simulink model "PMSM_NFLUX_v1_0"  (R2023b)
settings: Solver=FixedStepAuto  StartTime=0.0  StopTime=10.0  FixedStep=0.0001  RelTol=1e-3
values from neighbouring files (symbols this model uses):
  B = 8.0E-5    [PMSM_NFLUX.sldd]    (also in PMSM_NFLUX_backup_before_Simulink_RsStandstillID_20260617_154804.sldd; init_PMSM_NFLUX.m = single(8e-5))
  curr_d_ki = 35.0    [PMSM_NFLUX.sldd]    (also in PMSM_NFLUX_backup_before_Simulink_RsStandstillID_20260617_154804.sldd; init_PMSM_NFLUX.m = 35)
  curr_d_kp = 0.017    [PMSM_NFLUX.sldd]    (also in PMSM_NFLUX_backup_before_Simulink_RsStandstillID_20260617_154804.sldd; init_PMSM_NFLUX.m = 0.017)
  curr_q_ki = 35.0    [PMSM_NFLUX.sldd]    (also in PMSM_NFLUX_backup_before_Simulink_RsStandstillID_20260617_154804.sldd; init_PMSM_NFLUX.m = 35)
  curr_q_kp = 0.017    [PMSM_NFLUX.sldd]    (also in PMSM_NFLUX_backup_before_Simulink_RsStandstillID_20260617_154804.sldd; init_PMSM_NFLUX.m = 0.017)
  flux = 0.016884    [PMSM_NFLUX.sldd]    (also in PMSM_NFLUX_backup_before_Simulink_RsStandstillID_20260617_154804.sldd; init_PMSM_NFLUX.m = single(0.016884))
  Gamma = 100000.0    [PMSM_NFLUX.sldd]    (also in PMSM_NFLUX_backup_before_Simulink_RsStandstillID_20260617_154804.sldd; init_PMSM_NFLUX.m = single(100000.0))
  iq_handover = 0.4    [PMSM_NFLUX.sldd]    (also in PMSM_NFLUX_backup_before_Simulink_RsStandstillID_20260617_154804.sldd; init_PMSM_NFLUX.m = single(0.4))
  iq_ref_slew_down = 2.0    [PMSM_NFLUX.sldd]    (also in PMSM_NFLUX_backup_before_Simulink_RsStandstillID_20260617_154804.sldd; init_PMSM_NFLUX.m = single(2.0))
  iq_ref_slew_up = 5.0    [PMSM_NFLUX.sldd]    (also in PMSM_NFLUX_backup_before_Simulink_RsStandstillID_20260617_154804.sldd; init_PMSM_NFLUX.m = single(5.0))
  J = 7.5E-5    [PMSM_NFLUX.sldd]    (also in PMSM_NFLUX_backup_before_Simulink_RsStandstillID_20260617_154804.sldd; init_PMSM_NFLUX.m = single(75e-6))
  L = 0.00535    [PMSM_NFLUX.sldd]    (also in PMSM_NFLUX_backup_before_Simulink_RsStandstillID_20260617_154804.sldd; init_PMSM_NFLUX.m = single(0.00535))
  load_torque = 0.0    [PMSM_NFLUX.sldd]    (also in PMSM_NFLUX_backup_before_Simulink_RsStandstillID_20260617_154804.sldd; init_PMSM_NFLUX.m = single(0.0))
  LPF_K = 0.003    [PMSM_NFLUX.sldd]    (also in PMSM_NFLUX_backup_before_Simulink_RsStandstillID_20260617_154804.sldd; init_PMSM_NFLUX.m = single(0.003))
  PLL_Ki = 2500.0    [PMSM_NFLUX.sldd]    (also in PMSM_NFLUX_backup_before_Simulink_RsStandstillID_20260617_154804.sldd; init_PMSM_NFLUX.m = single(2500))
  PLL_Kp = 212.1    [PMSM_NFLUX.sldd]    (also in PMSM_NFLUX_backup_before_Simulink_RsStandstillID_20260617_154804.sldd; init_PMSM_NFLUX.m = single(212.1))
  PLL_OmegaLimit = 6283.18555    [PMSM_NFLUX.sldd]    (also in PMSM_NFLUX_backup_before_Simulink_RsStandstillID_20260617_154804.sldd; init_PMSM_NFLUX.m = single(2.0 * pi * 1000.0))
  Pn = 4.0    [PMSM_NFLUX.sldd]    (also in PMSM_NFLUX_backup_before_Simulink_RsStandstillID_20260617_154804.sldd; init_PMSM_NFLUX.m = single(4))
  PWM_HalfPeriod = 8000.0    [PMSM_NFLUX.sldd]    (also in PMSM_NFLUX_backup_before_Simulink_RsStandstillID_20260617_154804.sldd; init_PMSM_NFLUX.m = single(8000))
  Rs = 6.97    [PMSM_NFLUX.sldd]    (also in PMSM_NFLUX_backup_before_Simulink_RsStandstillID_20260617_154804.sldd; init_PMSM_NFLUX.m = single(6.97))
  spd_ki = 0.00165394868    [PMSM_NFLUX.sldd]    (also in PMSM_NFLUX_backup_before_Simulink_RsStandstillID_20260617_154804.sldd; init_PMSM_NFLUX.m = (B * speed_bw / Kt) * rpm_to_radps)
  spd_kp = 0.001550577    [PMSM_NFLUX.sldd]    (also in PMSM_NFLUX_backup_before_Simulink_RsStandstillID_20260617_154804.sldd; init_PMSM_NFLUX.m = (J * speed_bw / Kt) * rpm_to_radps)
  theta_handover_slew_limit = 5.0    [PMSM_NFLUX.sldd]    (also in PMSM_NFLUX_backup_before_Simulink_RsStandstillID_20260617_154804.sldd; init_PMSM_NFLUX.m = single(5.0))
  Tpwm = 16000.0    [PMSM_NFLUX.sldd]    (also in PMSM_NFLUX_backup_before_Simulink_RsStandstillID_20260617_154804.sldd; init_PMSM_NFLUX.m = 2 * PWM_HalfPeriod)
  Ts = 0.0001    [PMSM_NFLUX.sldd]    (also in PMSM_NFLUX_backup_before_Simulink_RsStandstillID_20260617_154804.sldd; init_PMSM_NFLUX.m = 0.0001)
  Udc = 24.0    [PMSM_NFLUX.sldd]    (also in PMSM_NFLUX_backup_before_Simulink_RsStandstillID_20260617_154804.sldd; init_PMSM_NFLUX.m = single(24.0))
undefined symbols (not defined in the file or in its folder): DiscIntNeverNeededParam, magnitude, sigbuilder_block
libraries: slpidlib x4, mcbplantlib x1, simulink x1, autolibpmsmexterior x1
(part 1 of 2)
settings Model: Creator=Administrator  LastModifiedBy=Kypuro

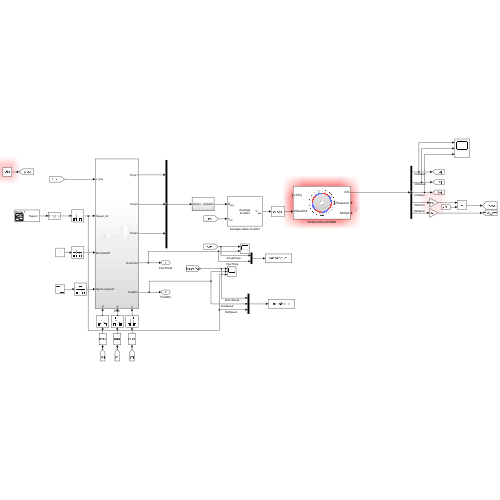
[thumbnail: Simulink's stored preview of the top-level diagram]
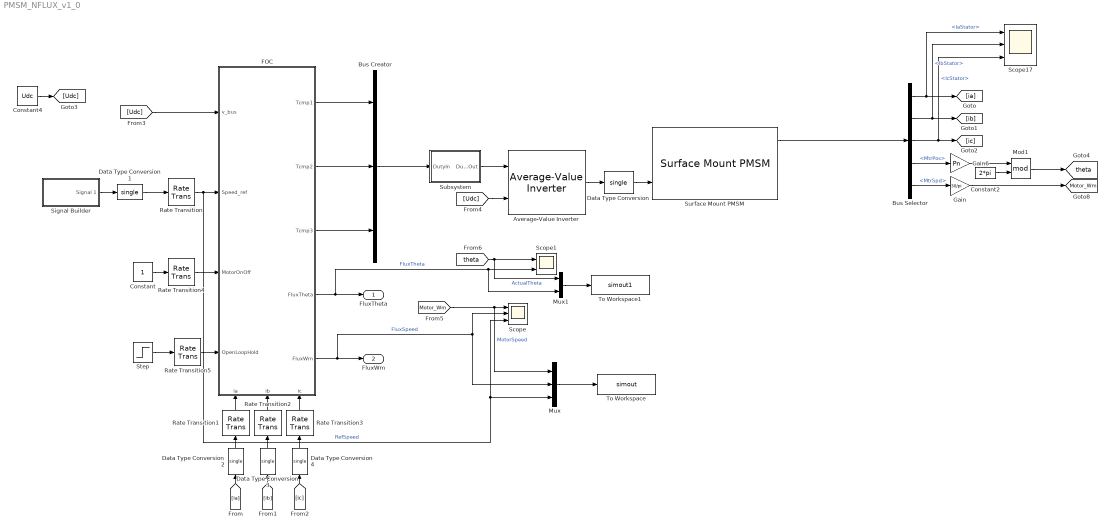
== system PMSM_NFLUX_v1_0 ==
  Average-Value Inverter : mcbplantlib/Average-Value Inverter
  Bus Creator : BusCreator  Inputs=3
  Bus Selector : BusSelector  OutputSignals=IaStator,IbStator,IcStator,MtrPos,MtrSpd
  Constant : Constant
  Constant2 : Constant  Value=2*pi  OutDataTypeStr=single
  Constant4 : Constant  Value=Udc  OutDataTypeStr=single
  Data Type Conversion{,1..4} (5 alike) : DataTypeConversion  OutDataTypeStr=single  SaturateOnIntegerOverflow=off  RndMeth=Floor
  FOC : Subsystem
      settings: PortSchema="{\"entries\":[{\"content\":{\"sides\":[{\"content\":{\"connectorIds\":[\"In1\",\"In2\",\"In3\",\"In4\"]},\"type\":\"ConnectorPlacement.EquallySpacedRectSide\",\"uuid\":\"15b5980d-6030-4553-a9ac-44e32f14a57a\"},{\"content\":{\"connectorIds\":[\"Out1\",\"Out2\",\"Out3\",\"Out4\",\"Out5\"],\"side\":\"RIGHT\"},\"type\":\"ConnectorPlacement.EquallySpacedRectSide\",\"uuid\":\"2f871f88-1192-4dfd-bfce-a65fb82dde08\"},{\"content\":{\"side\":\"TOP\"},\"type\":\"ConnectorPlacement.EquallySpacedRectSide\",\"uuid\":\"88b9ce00-4e74-42ee-98d0-7c23a9174907\"},{\"content\":{\"connectorIds\":[\"In5\",\"In6\",\"In7\"],\"side\":\"BOTTOM\"},\"type\":\"ConnectorPlacement.EquallySpacedRectSide\",\"uuid\":\"30df929a-c1ad-4497-8033-ccbdfa477756\"}]},\"type\":\"ConnectorPlacement.EquallySpacedConnector\",\"uuid\":\"d87cb52d-c5dd-4f26-b027-c0f882644c2a\"}],\"packageUris\":[\"http://schema.mathworks.com/mf0/Connector/R2020b\"],\"version\":\"1.0\"}"
  Gain : Gain  Gain=30/pi  OutDataTypeStr=single
  Gain6 : Gain  Gain=Pn  OutDataTypeStr=single
  Mod1 : Math  Operator=mod  OutputSignalType=real
  Mux : Mux  Inputs=3
  Mux1 : Mux  Inputs=2
  Rate Transition{,1..5} (6 alike) : RateTransition
  Scope : Scope  NumInputPorts=3
  Scope1 : Scope  NumInputPorts=2
  Scope17 : Scope  NumInputPorts=3
  Signal Builder : Subsystem  Tag=STV Subsys  LoadFcn=sigbuilder_block('load');  StartFcn=sigbuilder_block('start');  StopFcn=sigbuilder_block('stop');  ClipboardFcn=sigbuilder_block('clipboard');  mask(Sigbuilder block){tuvar=[0:10]}
      mask help: Simulink:masks:SigbuilderBlock_MD
      mask init:
      | if ~strcmp(get_param(bdroot(gcbh),'SimulationStatus'),'stopped') tuvar = sigbuilder_block('maskInit'); end
      settings: CopyFcn=sigbuilder_block('copy');  DeleteFcn=sigbuilder_block('delete');  ModelCloseFcn=sigbuilder_block('modelClose');  PreSaveFcn=sigbuilder_block('preSave');  PauseFcn=sigbuilder_block('pause');  ContinueFcn=sigbuilder_block('continue');  NameChangeFcn=sigbuilder_block('namechange');  OpenFcn=sigbuilder_block('open',[437.6 199.2 550.4 400 ]);  CloseFcn=sigbuilder_block('close');
      mask Display: plot(0, 0, 100, 100,[2, 2, 32, 32, 2], [68, 8, 8, 68, 68],[32, 2], [38, 38], [32, 19, 2],[53, 60, 44], [32, 17, 17, 2],[16, 16, 31, 31]);txt = getActiveGroup(gcbh);text(2, 100, txt,'verticalAlignment', 'top');
  Step : Step  Time=3  Before=1  After=0  SampleTime=0
  Subsystem : Subsystem
  Surface Mount PMSM : autolibpmsmexterior/Surface Mount PMSM  port_config=Torque  sim_type=Discrete  Ts=0.0001  FilePath=E:\Sandbox\Bauto\Work\surfacepmsm_motordata.m  P=Pn  Rs=Rs  Ldq_=L  KConstText=Permanent flux linkage constant (lambda_pm):  lambda_pm=flux  Ke=159.9771  Kt=1.323  mechanical=[J B load_torque]  idq0=[0 0]  theta_init=4/5  omega_init=0  KConst=flux  lambda_pm_calc=flux  RefBlkName='autolibpmsmexterior/Surface Mount PMSM'  aMode=1  Ldq="[0.0003752   0.0003752]"
      settings: LibrarySourceBlock=autolibemachines/Surface Mount PMSM
  To Workspace : ToWorkspace  VariableName=simout  SaveFormat=Timeseries  SampleTime=-1
  To Workspace1 : ToWorkspace  VariableName=simout1  SaveFormat=Timeseries  SampleTime=-1
  FluxTheta : Outport
  FluxWm : Outport  Port=2
  tag scope: Motor_Wm=global, theta=global
  wires:
  [Udc] -> FOC/1(v_bus)
  Rate Transition/1 -> Mux/3, Scope/3, FOC/2(Speed_ref)  "RefSpeed"
  Constant/1 -> Rate Transition4/1
  Step/1 -> Rate Transition5/1
  FOC/1(Tcmp1) -> Bus Creator/1
  FOC/2(Tcmp2) -> Bus Creator/2
  FOC/4(FluxTheta) -> Mux1/2, Scope1/2, FluxTheta/1  "FluxTheta"
  FOC/5(FluxWm) -> Scope/2, Mux/2, FluxWm/1  "FluxSpeed"
  Signal Builder/1(Signal 1) -> Data Type Conversion1/1
  Rate Transition1/1 -> FOC/5(ia)
  Rate Transition2/1 -> FOC/6(ib)
  Rate Transition3/1 -> FOC/7(ic)
  Rate Transition4/1 -> FOC/3(MotorOnOff)
  Rate Transition5/1 -> FOC/4(OpenLoopHold)
  Bus Creator/1 -> Subsystem/1(DutyIn)
  FOC/3(Tcmp3) -> Bus Creator/3
  Subsystem/1(DutyOut) -> Average-Value Inverter/1
  Constant4/1 -> [Udc]
  [Udc] -> Average-Value Inverter/2
  Average-Value Inverter/1 -> Data Type Conversion/1
  Surface Mount PMSM/1 -> Bus Selector/1
  Mod1/1 -> [theta]
  Gain6/1 -> Mod1/1
  Bus Selector/4 -> Gain6/1  "<MtrPos>"
  Bus Selector/3 -> [ic], Scope17/3  "<IcStator>"
  Constant2/1 -> Mod1/2
  Bus Selector/1 -> Scope17/1, [ia]  "<IaStator>"
  Bus Selector/2 -> [ib], Scope17/2  "<IbStator>"
  Data Type Conversion/1 -> Surface Mount PMSM/2
  Data Type Conversion1/1 -> Rate Transition/1
  Data Type Conversion2/1 -> Rate Transition1/1
  [ia] -> Data Type Conversion2/1
  Data Type Conversion3/1 -> Rate Transition2/1
  [ib] -> Data Type Conversion3/1
  Data Type Conversion4/1 -> Rate Transition3/1
  [ic] -> Data Type Conversion4/1
  [Motor_Wm] -> Mux/1, Scope/1  "MotorSpeed"
  [theta] -> Mux1/1, Scope1/1  "ActualTheta"
  Gain/1 -> [Motor_Wm]
  Bus Selector/5 -> Gain/1  "<MtrSpd>"
  Mux/1 -> To Workspace/1
  Mux1/1 -> To Workspace1/1

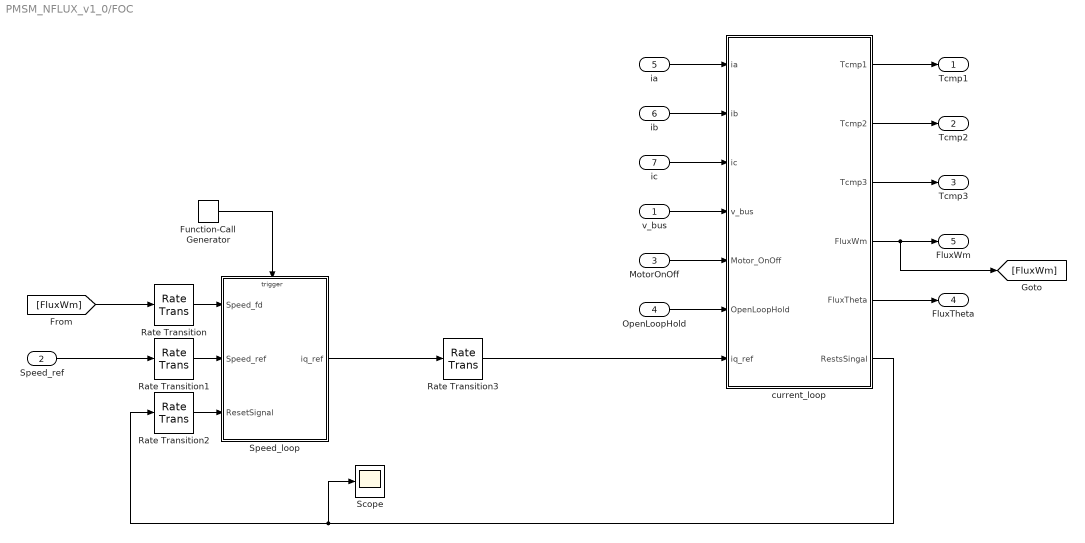
== system PMSM_NFLUX_v1_0/FOC ==
  v_bus : Inport
  Speed_ref : Inport  Port=2
  MotorOnOff : Inport  Port=3
  OpenLoopHold : Inport  Port=4
  ia : Inport  Port=5
  ib : Inport  Port=6
  ic : Inport  Port=7
  Function-Call Generator : simulink/Ports & Subsystems/Function-Call Generator  sample_time=1e-3  numberOfIterations=1  DisallowWideOutput=off
  Rate Transition{,1..3} (4 alike) : RateTransition
  Scope : Scope
  Speed_loop : Subsystem
  current_loop : Subsystem
  Tcmp1 : Outport
  Tcmp2 : Outport  Port=2
  Tcmp3 : Outport  Port=3
  FluxTheta : Outport  Port=4
  FluxWm : Outport  Port=5
  wires:
  Rate Transition2/1 -> Speed_loop/3(ResetSignal)
  current_loop/3(Tcmp3) -> Tcmp3/1
  Rate Transition1/1 -> Speed_loop/2(Speed_ref)
  Rate Transition/1 -> Speed_loop/1(Speed_fd)
  Function-Call Generator/1 -> Speed_loop/Trigger
  ic/1 -> current_loop/3(ic)
  OpenLoopHold/1 -> current_loop/6(OpenLoopHold)
  current_loop/4(FluxWm) -> FluxWm/1, [FluxWm]
  current_loop/1(Tcmp1) -> Tcmp1/1
  ia/1 -> current_loop/1(ia)
  MotorOnOff/1 -> current_loop/5(Motor_OnOff)
  Speed_ref/1 -> Rate Transition1/1
  ib/1 -> current_loop/2(ib)
  Speed_loop/1(iq_ref) -> Rate Transition3/1
  Rate Transition3/1 -> current_loop/7(iq_ref)
  current_loop/2(Tcmp2) -> Tcmp2/1
  current_loop/5(FluxTheta) -> FluxTheta/1
  current_loop/6(RestsSingal) -> Scope/1, Rate Transition2/1
  v_bus/1 -> current_loop/4(v_bus)
  [FluxWm] -> Rate Transition/1

== system PMSM_NFLUX_v1_0/Signal Builder ==
  Demux : Demux  Tag=STV Demux  Outputs=1
      settings: DisplayOption=none
  FromWs : FromWorkspace  Tag=STV FromWs  VariableName=tuvar
      SigBuilderData=|
      | common.afterFinalStr = 'Extrapolate'
      | common.sampleTime = 0
      | dataSet.timeRange = [0 10]
      | dataSet.name = 'Group 1'
      | sbobj.Groups.Name = 'Group 1'
      | sbobj.Groups.Signals.Name = 'Signal 1'
      | sbobj.Groups.Signals.XData = [0 4 4 7 7 10]
      | sbobj.Groups.Signals.YData = [680 680 1020 1020 1200 1200]
  Signal 1 : Outport  Tag=STV Outport
  wires:
  Demux/1 -> Signal 1/1
  FromWs/1 -> Demux/1

== system PMSM_NFLUX_v1_0/Subsystem ==
  DutyIn : Inport
  Constant : Constant  Value=0.5  SampleTime=-1
  Gain : Gain  Gain=1/PWM_HalfPeriod  ParamDataTypeStr=single
  Gain1 : Gain  Gain=-1
  Sum : Sum  Inputs=|+-
  Sum1 : Sum  Inputs=|++
  DutyOut : Outport
  wires:
  Sum/1 -> Gain1/1
  Constant/1 -> Sum1/2, Sum/2
  DutyIn/1 -> Gain/1
  Gain1/1 -> Sum1/1
  Sum1/1 -> DutyOut/1
  Gain/1 -> Sum/1

== system PMSM_NFLUX_v1_0/FOC/Speed_loop ==
  Speed_fd : Inport  OutDataTypeStr=single  PortDimensions=1
  Speed_ref : Inport  Port=2  OutDataTypeStr=single  PortDimensions=1
  ResetSignal : Inport  Port=3
  Trigger : TriggerPort  TriggerType=function-call  VariantControl=(inherit)  PortDimensions=1
  PID Controller3 : slpidlib/PID Controller  Controller=PI  Form=Parallel  TimeDomain=Discrete-time  UseExternalTs=off  SampleTime=-1  IntegratorMethod=Forward Euler  FilterMethod=Forward Euler  ControllerParametersSource=internal  P=spd_kp  I=spd_ki  UseKiTs=off  D=0  N=100  UseFilter=on  TunerSelectOption=Transfer Function Based (PID Tuner App)  InitialConditionSource=internal  InitialConditionForIntegrator=0  InitialConditionForFilter=0  DifferentiatorICPrevScaledInput=0  ExternalReset=rising  TrackingMode=off  Kt=1  LimitOutput=on  SatLimitsSource=internal  UpperSaturationLimit=3  LowerSaturationLimit=-3  LinearizeAsGain=on  AntiWindupMode=clamping  Kb=0.013  LimitIntegrator=off  UpperIntegratorSaturationLimit=inf  LowerIntegratorSaturationLimit=-inf  PGainOutDataTypeStr=single  PProdOutDataTypeStr=single  POutMin=[]  POutMax=[]  IGainOutDataTypeStr=single  IProdOutDataTypeStr=single  IOutMin=[]  IOutMax=[]  DOutMin=[]  DOutMax=[]  NOutMin=[]  NOutMax=[]  SumOutDataTypeStr=single  SumOutMin=[]  SumOutMax=[]  SaturationOutDataTypeStr=single  SaturationOutMin=[]  SaturationOutMax=[]  PParamMin=[]  PParamMax=[]  IParamMin=[]  IParamMax=[]  DParamMin=[]  DParamMax=[]  NParamMin=[]  NParamMax=[]  KbParamMin=[]  KbParamMax=[]  KtParamMin=[]  KtParamMax=[]  KbOutMin=[]  KbOutMax=[]  KtOutMin=[]  KtOutMax=[]  IntegratorOutMin=[]  IntegratorOutMax=[]  FilterOutMin=[]  FilterOutMax=[]  SumI1OutMin=[]  SumI1OutMax=[]  SumI2OutMin=[]  SumI2OutMax=[]  SumI3OutMin=[]  SumI3OutMax=[]  SumI4OutMin=[]  SumI4OutMax=[]  SumDOutMin=[]  SumDOutMax=[]  DifferentiatorOutMin=[]  DifferentiatorOutMax=[]  FilterDiffOutCoefMin=[]  FilterDiffOutCoefMax=[]  ReciprocalOutMin=[]  ReciprocalOutMax=[]  SumDenOutMin=[]  SumDenOutMax=[]  SumNumOutMin=[]  SumNumOutMax=[]  DivideOutMin=[]  DivideOutMax=[]  UdiffTsProdOutMin=[]  UdiffTsProdOutMax=[]  NTsProdOutMin=[]  NTsProdOutMax=[]  UintegralTsProdOutMin=[]  UintegralTsProdOutMax=[]  UngainTsProdOutMin=[]  UngainTsProdOutMax=[]  ClampingZeroOutDataTypeStr=Inherit: Inherit via back propagation  ClampingZeroOutMin=[]  ClampingZeroOutMax=[]  FilterDenConstantOutDataTypeStr=Inherit: Inherit via back propagation  FilterDenConstantOutMin=[]  FilterDenConstantOutMax=[]  PCopyOutDataTypeStr=Inherit: Inherit via back propagation  PCopyOutMin=[]  PCopyOutMax=[]  NCopyOutDataTypeStr=Inherit: Inherit via back propagation  NCopyOutMin=[]  NCopyOutMax=[]  IntegratorContinuousStateAttributes=''  IntegratorStateMustResolveToSignalObject=off  IntegratorRTWStateStorageClass=Auto  FilterContinuousStateAttributes=''  FilterStateMustResolveToSignalObject=off  FilterRTWStateStorageClass=Auto  ParallelPVariant=InternalParameters  IdealPVariant=Disabled  IVariant=InternalParameters  DVariant=Disabled  IntegratorVariant=Discrete  SatVariant=Enabled  AWVariant=DiscClampingParallel  PCopyVariant=Disabled  TRVariant=Disabled  FdbkBlocksVariant=Forward  IdealPFdbkVariant=Disabled  SatFdbkVariant=Disabled  DerivativeFilterVariant=Disabled  NVariant=Disabled  NCopyVariant=Disabled_SignalSpec  FilterICVariant=Disabled  IntegratorICVariant=InternalICs  ExternalResetVariant=ExternalReset  TRSumVariant=Passthrough  SumFdbkVariant=Disabled  SumVariant=Sum_PI  TsampFilterVariant=InternalTs  TsampNgainVariant=Passthrough  TsampIntegralVariant=Disabled_SignalSpec  ExternalSaturationOutDataTypeStr=single
  Scope : Scope
  Sum2 : Sum  Inputs=|+-  OutDataTypeStr=single  AccumDataTypeStr=single
  iq_ref : Outport
  wires:
  Sum2/1 -> Scope/1, PID Controller3/1
  Speed_ref/1 -> Sum2/1
  Speed_fd/1 -> Sum2/2
  PID Controller3/1 -> iq_ref/1
  ResetSignal/1 -> PID Controller3/2

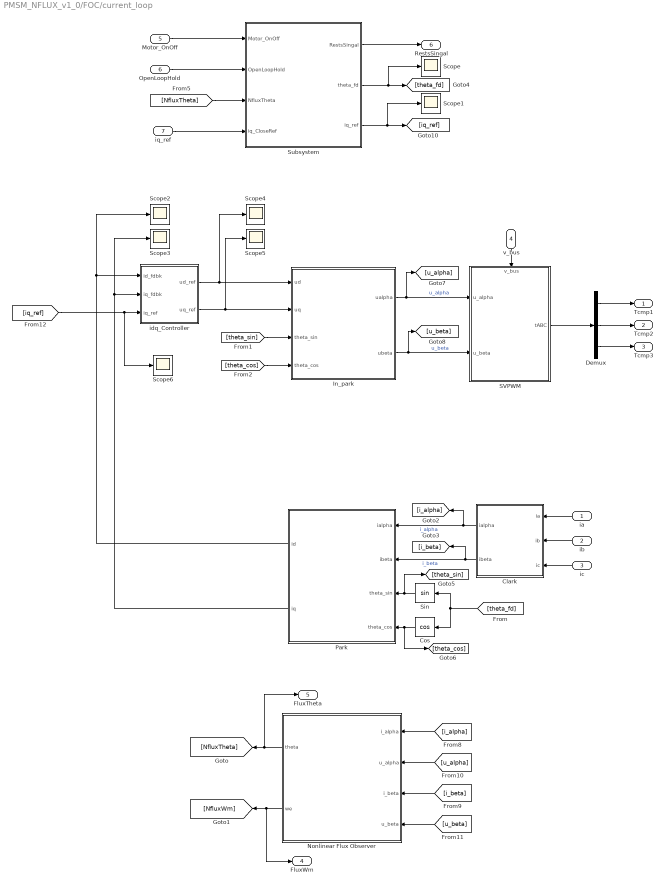
== system PMSM_NFLUX_v1_0/FOC/current_loop ==
  ia : Inport
  ib : Inport  Port=2
  ic : Inport  Port=3
  v_bus : Inport  Port=4
  Motor_OnOff : Inport  Port=5
  OpenLoopHold : Inport  Port=6
  iq_ref : Inport  Port=7
  Clark : Subsystem  TreatAsAtomicUnit=on
  Cos : Trigonometry  Operator=cos
  Demux : Demux  Outputs=3
  In_park : Subsystem  TreatAsAtomicUnit=on
  Nonlinear Flux Observer : Subsystem
  Park : Subsystem  TreatAsAtomicUnit=on
  SVPWM : Subsystem  TreatAsAtomicUnit=on
      settings: PortSchema="{\"entries\":[{\"content\":{\"sides\":[{\"content\":{\"connectorIds\":[\"In1\",\"In2\"]},\"type\":\"ConnectorPlacement.EquallySpacedRectSide\",\"uuid\":\"4b32ca5b-ab58-435f-bafc-1a0f46196043\"},{\"content\":{\"connectorIds\":[\"Out1\"],\"side\":\"RIGHT\"},\"type\":\"ConnectorPlacement.EquallySpacedRectSide\",\"uuid\":\"0d0dcd90-817b-446f-b64d-13f641f634d9\"},{\"content\":{\"connectorIds\":[\"In3\"],\"side\":\"TOP\"},\"type\":\"ConnectorPlacement.EquallySpacedRectSide\",\"uuid\":\"44cad929-24bb-40f4-a976-89e6181a2a02\"}]},\"type\":\"ConnectorPlacement.EquallySpacedConnector\",\"uuid\":\"e76fe955-91e8-40d5-8302-6240a99fd5a2\"}],\"packageUris\":[\"http://schema.mathworks.com/mf0/Connector/R2020b\"],\"version\":\"1.0\"}"
  Scope{,1..6} (7 alike) : Scope
  Sin : Trigonometry
  Subsystem : Subsystem
  idq_Controller : Subsystem
  Tcmp1 : Outport
  Tcmp2 : Outport  Port=2
  Tcmp3 : Outport  Port=3
  FluxWm : Outport  Port=4
  FluxTheta : Outport  Port=5
  RestsSingal : Outport  Port=6
  wires:
  Cos/1 -> [theta_cos], Park/4(theta_cos)
  Clark/2(ibeta) -> [i_beta], Park/2(ibeta)  "i_beta"
  In_park/2(ubeta) -> [u_beta], SVPWM/2(u_beta)  "u_beta"
  [theta_fd] -> Cos/1, Sin/1
  Nonlinear Flux Observer/2(we) -> FluxWm/1, [NfluxWm]
  Sin/1 -> [theta_sin], Park/3(theta_sin)
  [i_beta] -> Nonlinear Flux Observer/3(i_beta)
  ic/1 -> Clark/3(ic)
  [theta_sin] -> In_park/3(theta_sin)
  In_park/1(ualpha) -> SVPWM/1(u_alpha), [u_alpha]  "u_alpha"
  Nonlinear Flux Observer/1(theta) -> FluxTheta/1, [NfluxTheta]
  idq_Controller/1(ud_ref) -> Scope4/1, In_park/1(ud)
  Clark/1(ialpha) -> [i_alpha], Park/1(ialpha)  "i_alpha"
  Park/2(iq) -> Scope3/1, idq_Controller/2(iq_fdbk)
  Park/1(id) -> Scope2/1, idq_Controller/1(id_fdbk)
  Demux/1 -> Tcmp1/1
  idq_Controller/2(uq_ref) -> Scope5/1, In_park/2(uq)
  Demux/3 -> Tcmp3/1
  ib/1 -> Clark/2(ib)
  ia/1 -> Clark/1(ia)
  SVPWM/1(tABC) -> Demux/1
  [iq_ref] -> Scope6/1, idq_Controller/3(iq_ref)
  [i_alpha] -> Nonlinear Flux Observer/1(i_alpha)
  [theta_cos] -> In_park/4(theta_cos)
  v_bus/1 -> SVPWM/3(v_bus)
  [u_beta] -> Nonlinear Flux Observer/4(u_beta)
  [u_alpha] -> Nonlinear Flux Observer/2(u_alpha)
  Demux/2 -> Tcmp2/1
  Subsystem/2(theta_fd) -> Scope/1, [theta_fd]
  Motor_OnOff/1 -> Subsystem/1(Motor_OnOff)
  OpenLoopHold/1 -> Subsystem/2(OpenLoopHold)
  [NfluxTheta] -> Subsystem/3(NfluxTheta)
  iq_ref/1 -> Subsystem/4(iq_CloseRef)
  Subsystem/1(RestsSingal) -> RestsSingal/1
  Subsystem/3(iq_ref) -> Scope1/1, [iq_ref]

== system PMSM_NFLUX_v1_0/FOC/current_loop/Clark ==
  note: ialpha = ia*2/3-(ib+ic)/3;
      | ibeta = (ib-ic)*sqrt(3)/3;
  ia : Inport  OutDataTypeStr=single
  ib : Inport  Port=2  OutDataTypeStr=single
  ic : Inport  Port=3  OutDataTypeStr=single
  Add : Sum  OutDataTypeStr=single  AccumDataTypeStr=single
  Add1 : Sum  Inputs=+-  OutDataTypeStr=single  AccumDataTypeStr=single
  Add2 : Sum  Inputs=+-  OutDataTypeStr=single  AccumDataTypeStr=single
  Gain : Gain  Gain=2/3  ParamDataTypeStr=single
  Gain1 : Gain  Gain=1/3  ParamDataTypeStr=single
  Gain2 : Gain  Gain=sqrt(3)/3  ParamDataTypeStr=single
  ialpha : Outport  OutDataTypeStr=single
  ibeta : Outport  Port=2  OutDataTypeStr=single
  wires:
  ia/1 -> Gain/1
  ib/1 -> Add2/1, Add/1
  ic/1 -> Add2/2, Add/2
  Add/1 -> Gain1/1
  Gain/1 -> Add1/1
  Gain1/1 -> Add1/2
  Add1/1 -> ialpha/1
  Add2/1 -> Gain2/1
  Gain2/1 -> ibeta/1

== system PMSM_NFLUX_v1_0/FOC/current_loop/In_park ==
  note: Valpha = ud*cos(theta) - uq*sin(theta);
      | Vbeta = ud*sin(theta) + uq*cos(theta);
  ud : Inport
  uq : Inport  Port=2
  theta_sin : Inport  Port=3
  theta_cos : Inport  Port=4
  Add : Sum  Inputs=+-
  Add1 : Sum
  Product{,1..3} (4 alike) : Product
  ualpha : Outport
  ubeta : Outport  Port=2
  wires:
  Add/1 -> ualpha/1
  ud/1 -> Product2/1, Product/1
  theta_cos/1 -> Product/2, Product3/2
  Product/1 -> Add/1
  uq/1 -> Product3/1, Product1/1
  theta_sin/1 -> Product2/2, Product1/2
  Product1/1 -> Add/2
  Product2/1 -> Add1/1
  Product3/1 -> Add1/2
  Add1/1 -> ubeta/1

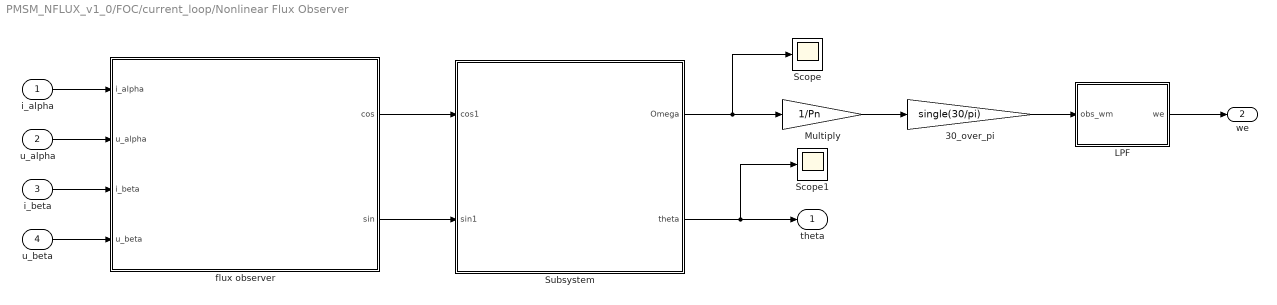
== system PMSM_NFLUX_v1_0/FOC/current_loop/Nonlinear Flux Observer ==
  i_alpha : Inport  OutDataTypeStr=single  PortDimensions=1
  u_alpha : Inport  Port=2  OutDataTypeStr=single  PortDimensions=1
  i_beta : Inport  Port=3  OutDataTypeStr=single  PortDimensions=1
  u_beta : Inport  Port=4  OutDataTypeStr=single  PortDimensions=1
  30_over_pi : Gain  Gain=single(30/pi)
  LPF : Subsystem
  Multiply : Gain  Gain=1/Pn
  Scope : Scope
  Scope1 : Scope
  Subsystem : Subsystem
  flux observer : Subsystem
  theta : Outport  OutDataTypeStr=single
  we : Outport  Port=2
  wires:
  u_beta/1 -> flux observer/4(u_beta)
  LPF/1(we) -> we/1
  flux observer/2(sin) -> Subsystem/2(sin1)
  30_over_pi/1 -> LPF/1(obs_wm)
  u_alpha/1 -> flux observer/2(u_alpha)
  i_alpha/1 -> flux observer/1(i_alpha)
  Multiply/1 -> 30_over_pi/1
  i_beta/1 -> flux observer/3(i_beta)
  Subsystem/2(theta) -> Scope1/1, theta/1
  flux observer/1(cos) -> Subsystem/1(cos1)
  Subsystem/1(Omega) -> Scope/1, Multiply/1

== system PMSM_NFLUX_v1_0/FOC/current_loop/Park ==
  note: id = ialpha*cos(theta)+ibeta*sin(theta);
      | iq = -ialpha*sin(theta)+ibeta*cos(theta);
  ialpha : Inport  OutDataTypeStr=single
  ibeta : Inport  Port=2  OutDataTypeStr=single
  theta_sin : Inport  Port=3  OutDataTypeStr=single
  theta_cos : Inport  Port=4  OutDataTypeStr=single
  Add : Sum  OutDataTypeStr=single  AccumDataTypeStr=single
  Add1 : Sum  Inputs=-+  OutDataTypeStr=single  AccumDataTypeStr=single
  Product{,1..3} (4 alike) : Product  OutDataTypeStr=single
  id : Outport  OutDataTypeStr=single
  iq : Outport  Port=2  OutDataTypeStr=single
  wires:
  ialpha/1 -> Product2/1, Product/1
  theta_cos/1 -> Product3/2, Product/2
  ibeta/1 -> Product3/1, Product1/1
  theta_sin/1 -> Product2/2, Product1/2
  Product/1 -> Add/1
  Product1/1 -> Add/2
  Add/1 -> id/1
  Product2/1 -> Add1/1
  Product3/1 -> Add1/2
  Add1/1 -> iq/1

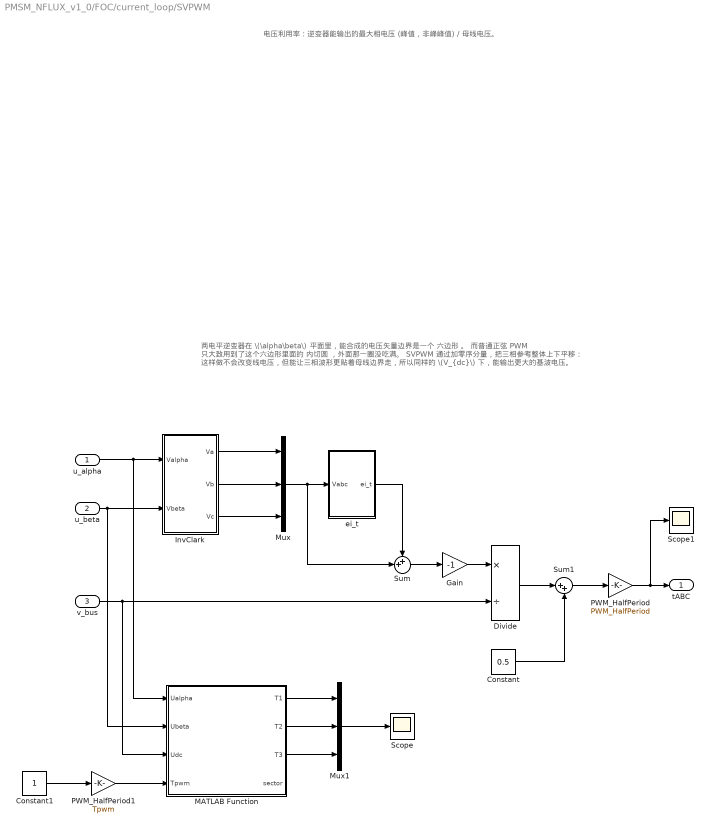
== system PMSM_NFLUX_v1_0/FOC/current_loop/SVPWM ==
  note: 电压利用率：逆变器能输出的最大相电压 (峰值，非峰峰值) / 母线电压。
  note: 两电平逆变器在 \(\alpha\beta\) 平面里，能合成的电压矢量边界是一个 六边形 。
      | 而普通正弦 PWM 只大致用到了这个六边形里面的 内切圆 ，外面那一圈没吃满。
      | SVPWM 通过加零序分量，把三相参考整体上下平移：
      | 这样做不会改变线电压，但能让三相波形更贴着母线边界走，所以同样的 \(V_{dc}\) 下，能输出更大的基波电压。
  u_alpha : Inport  OutDataTypeStr=single
  u_beta : Inport  Port=2  OutDataTypeStr=single
  v_bus : Inport  Port=3  OutDataTypeStr=single
  Constant : Constant  Value=0.5  OutDataTypeStr=single
  Constant1 : Constant
  Divide : Product  Inputs=*/  OutDataTypeStr=single
  Gain : Gain  Gain=-1  OutDataTypeStr=single
  InvClark : Subsystem
  MATLAB Function : MATLAB Function  TreatAsAtomicUnit=on
  Mux : Mux  Inputs=3
  Mux1 : Mux  Inputs=3
  PWM_HalfPeriod : Gain  Gain=PWM_HalfPeriod  OutDataTypeStr=single
  PWM_HalfPeriod1 : Gain  Gain=Tpwm  OutDataTypeStr=single
  Scope : Scope
  Scope1 : Scope
  Sum : Sum  Inputs=++|  OutDataTypeStr=single
  Sum1 : Sum  Inputs=|++  OutDataTypeStr=single
  ei_t : Subsystem
  tABC : Outport  OutDataTypeStr=single
  wires:
  u_alpha/1 -> MATLAB Function/1(Ualpha), InvClark/1(Valpha)
  u_beta/1 -> MATLAB Function/2(Ubeta), InvClark/2(Vbeta)
  ei_t/1(ei_t) -> Sum/1
  InvClark/1(Va) -> Mux/1
  InvClark/2(Vb) -> Mux/2
  InvClark/3(Vc) -> Mux/3
  Sum/1 -> Gain/1
  Mux/1 -> Sum/2, ei_t/1(Vabc)
  Divide/1 -> Sum1/1
  Constant/1 -> Sum1/2
  Sum1/1 -> PWM_HalfPeriod/1
  PWM_HalfPeriod/1 -> Scope1/1, tABC/1
  v_bus/1 -> MATLAB Function/3(Udc), Divide/2
  Gain/1 -> Divide/1
  PWM_HalfPeriod1/1 -> MATLAB Function/4(Tpwm)
  Constant1/1 -> PWM_HalfPeriod1/1
  MATLAB Function/1(T1) -> Mux1/1
  MATLAB Function/2(T2) -> Mux1/2
  MATLAB Function/3(T3) -> Mux1/3
  Mux1/1 -> Scope/1

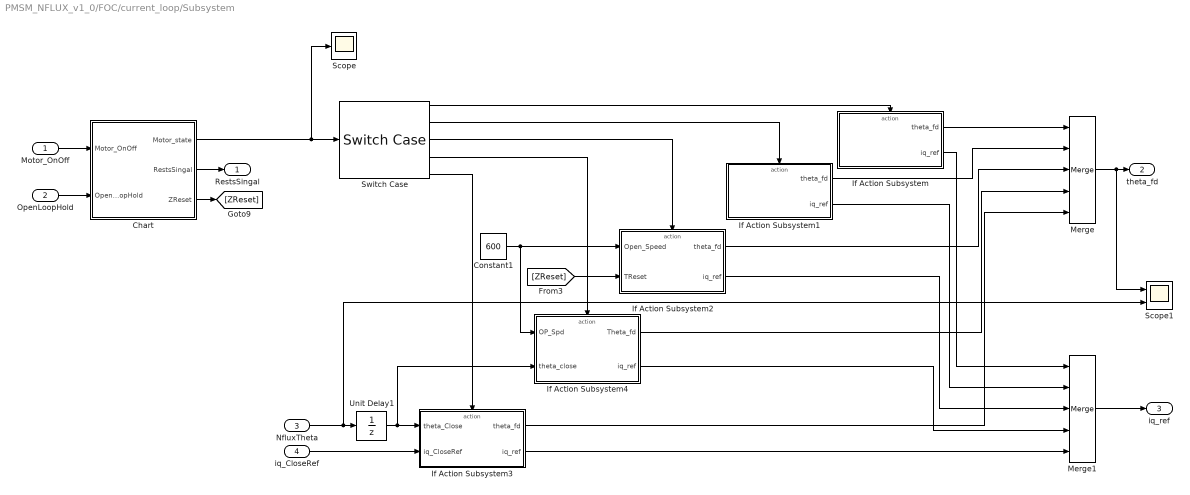
== system PMSM_NFLUX_v1_0/FOC/current_loop/Subsystem ==
  Motor_OnOff : Inport
  OpenLoopHold : Inport  Port=2
  NfluxTheta : Inport  Port=3
  iq_CloseRef : Inport  Port=4
  Chart : Stateflow chart  TreatAsAtomicUnit=on
  Constant1 : Constant  Value=600  OutDataTypeStr=int32
  If Action Subsystem : Subsystem  TreatAsAtomicUnit=on
  If Action Subsystem1 : Subsystem  TreatAsAtomicUnit=on
  If Action Subsystem2 : Subsystem  TreatAsAtomicUnit=on
  If Action Subsystem3 : Subsystem  TreatAsAtomicUnit=on
  If Action Subsystem4 : Subsystem  TreatAsAtomicUnit=on
  Merge : Merge  Inputs=5
  Merge1 : Merge  Inputs=5
  Scope : Scope
  Scope1 : Scope  NumInputPorts=2
  Switch Case : SwitchCase  CaseConditions={1,2,3,4,5}  ShowDefaultCase=off
  Unit Delay1 : UnitDelay  SampleTime=-1  HasFrameUpgradeWarning=on
  RestsSingal : Outport
  theta_fd : Outport  Port=2
  iq_ref : Outport  Port=3
  wires:
  Switch Case/5 -> If Action Subsystem3/Action
  [ZReset] -> If Action Subsystem2/2(TReset)
  Switch Case/1 -> If Action Subsystem/Action
  Merge1/1 -> iq_ref/1
  If Action Subsystem4/1(Theta_fd) -> Merge/4
  Chart/1(Motor_state) -> Scope/1, Switch Case/1
  If Action Subsystem3/1(theta_fd) -> Merge/5
  Chart/3(ZReset) -> [ZReset]
  iq_CloseRef/1 -> If Action Subsystem3/2(iq_CloseRef)
  Switch Case/2 -> If Action Subsystem1/Action
  If Action Subsystem2/1(theta_fd) -> Merge/3
  If Action Subsystem/1(theta_fd) -> Merge/1
  Constant1/1 -> If Action Subsystem4/1(OP_Spd), If Action Subsystem2/1(Open_Speed)
  If Action Subsystem1/1(theta_fd) -> Merge/2
  Switch Case/4 -> If Action Subsystem4/Action
  Switch Case/3 -> If Action Subsystem2/Action
  If Action Subsystem/2(iq_ref) -> Merge1/1
  If Action Subsystem2/2(iq_ref) -> Merge1/3
  Unit Delay1/1 -> If Action Subsystem4/2(theta_close), If Action Subsystem3/1(theta_Close)
  Chart/2(RestsSingal) -> RestsSingal/1
  If Action Subsystem1/2(iq_ref) -> Merge1/2
  If Action Subsystem3/2(iq_ref) -> Merge1/5
  If Action Subsystem4/2(iq_ref) -> Merge1/4
  Motor_OnOff/1 -> Chart/1(Motor_OnOff)
  Merge/1 -> Scope1/1, theta_fd/1
  OpenLoopHold/1 -> Chart/2(OpenLoopHold)
  NfluxTheta/1 -> Scope1/2, Unit Delay1/1

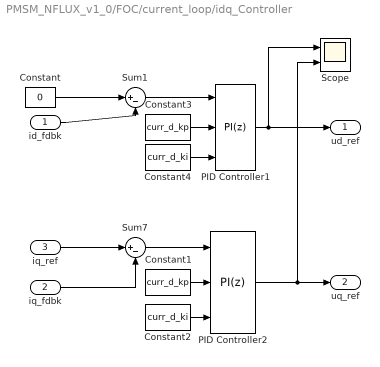
== system PMSM_NFLUX_v1_0/FOC/current_loop/idq_Controller ==
  id_fdbk : Inport  OutDataTypeStr=single
  iq_fdbk : Inport  Port=2  OutDataTypeStr=single
  iq_ref : Inport  Port=3  OutDataTypeStr=single
  Constant : Constant  Value=0  OutDataTypeStr=single
  Constant1 : Constant  Value=curr_d_kp  OutDataTypeStr=single
  Constant2 : Constant  Value=curr_d_ki  OutDataTypeStr=single
  Constant3 : Constant  Value=curr_d_kp  OutDataTypeStr=single
  Constant4 : Constant  Value=curr_d_ki  OutDataTypeStr=single
  PID Controller1 : slpidlib/PID Controller  Controller=PI  Form=Parallel  TimeDomain=Discrete-time  UseExternalTs=off  SampleTime=-1  IntegratorMethod=Forward Euler  FilterMethod=Forward Euler  ControllerParametersSource=external  P=curr_d_kp  I=curr_d_ki  UseKiTs=off  D=0  N=100  UseFilter=on  TunerSelectOption=Transfer Function Based (PID Tuner App)  InitialConditionSource=internal  InitialConditionForIntegrator=0  InitialConditionForFilter=0  DifferentiatorICPrevScaledInput=0  ExternalReset=none  TrackingMode=off  Kt=1  LimitOutput=on  SatLimitsSource=internal  UpperSaturationLimit=24*0.9/sqrt(3)  LowerSaturationLimit=-24*0.9/sqrt(3)  LinearizeAsGain=on  AntiWindupMode=clamping  Kb=1  LimitIntegrator=off  UpperIntegratorSaturationLimit=inf  LowerIntegratorSaturationLimit=-inf  PGainOutDataTypeStr=single  PProdOutDataTypeStr=single  POutMin=[]  POutMax=[]  IGainOutDataTypeStr=int16  IProdOutDataTypeStr=int16  IOutMin=[]  IOutMax=[]  DOutMin=[]  DOutMax=[]  NOutMin=[]  NOutMax=[]  SumOutDataTypeStr=single  SumOutMin=[]  SumOutMax=[]  SaturationOutDataTypeStr=single  SaturationOutMin=[]  SaturationOutMax=[]  PParamMin=[]  PParamMax=[]  IParamMin=[]  IParamMax=[]  DParamMin=[]  DParamMax=[]  NParamMin=[]  NParamMax=[]  KbParamMin=[]  KbParamMax=[]  KtParamMin=[]  KtParamMax=[]  KbOutMin=[]  KbOutMax=[]  KtOutMin=[]  KtOutMax=[]  IntegratorOutMin=[]  IntegratorOutMax=[]  FilterOutMin=[]  FilterOutMax=[]  SumI1OutMin=[]  SumI1OutMax=[]  SumI2OutMin=[]  SumI2OutMax=[]  SumI3OutMin=[]  SumI3OutMax=[]  SumI4OutMin=[]  SumI4OutMax=[]  SumDOutMin=[]  SumDOutMax=[]  DifferentiatorOutMin=[]  DifferentiatorOutMax=[]  FilterDiffOutCoefMin=[]  FilterDiffOutCoefMax=[]  ReciprocalOutMin=[]  ReciprocalOutMax=[]  SumDenOutMin=[]  SumDenOutMax=[]  SumNumOutMin=[]  SumNumOutMax=[]  DivideOutMin=[]  DivideOutMax=[]  UdiffTsProdOutMin=[]  UdiffTsProdOutMax=[]  NTsProdOutMin=[]  NTsProdOutMax=[]  UintegralTsProdOutMin=[]  UintegralTsProdOutMax=[]  UngainTsProdOutMin=[]  UngainTsProdOutMax=[]  ClampingZeroOutDataTypeStr=Inherit: Inherit via back propagation  ClampingZeroOutMin=[]  ClampingZeroOutMax=[]  FilterDenConstantOutDataTypeStr=Inherit: Inherit via back propagation  FilterDenConstantOutMin=[]  FilterDenConstantOutMax=[]  PCopyOutDataTypeStr=Inherit: Inherit via back propagation  PCopyOutMin=[]  PCopyOutMax=[]  NCopyOutDataTypeStr=Inherit: Inherit via back propagation  NCopyOutMin=[]  NCopyOutMax=[]  IntegratorContinuousStateAttributes=''  IntegratorStateMustResolveToSignalObject=off  IntegratorRTWStateStorageClass=Auto  FilterContinuousStateAttributes=''  FilterStateMustResolveToSignalObject=off  FilterRTWStateStorageClass=Auto  ParallelPVariant=ExternalParameters  IdealPVariant=Disabled  IVariant=ExternalParameters  DVariant=Disabled  IntegratorVariant=Discrete  SatVariant=Enabled  AWVariant=DiscClampingParallel  PCopyVariant=Disabled  TRVariant=Disabled  FdbkBlocksVariant=Forward  IdealPFdbkVariant=Disabled  SatFdbkVariant=Disabled  DerivativeFilterVariant=Disabled  NVariant=Disabled  NCopyVariant=Disabled_SignalSpec  FilterICVariant=Disabled  IntegratorICVariant=InternalICs  ExternalResetVariant=Disabled  TRSumVariant=Passthrough  SumFdbkVariant=Disabled  SumVariant=Sum_PI  TsampFilterVariant=InternalTs  TsampNgainVariant=Passthrough  TsampIntegralVariant=Disabled_SignalSpec  ExternalSaturationOutDataTypeStr=Inherit: Same as second input
  PID Controller2 : slpidlib/PID Controller  Controller=PI  Form=Parallel  TimeDomain=Discrete-time  UseExternalTs=off  SampleTime=-1  IntegratorMethod=Forward Euler  FilterMethod=Forward Euler  ControllerParametersSource=external  P=curr_q_kp  I=curr_q_ki  UseKiTs=off  D=0  N=100  UseFilter=on  TunerSelectOption=Transfer Function Based (PID Tuner App)  InitialConditionSource=internal  InitialConditionForIntegrator=0  InitialConditionForFilter=0  DifferentiatorICPrevScaledInput=0  ExternalReset=none  TrackingMode=off  Kt=1  LimitOutput=on  SatLimitsSource=internal  UpperSaturationLimit=24*0.9/sqrt(3)  LowerSaturationLimit=-24*0.9/sqrt(3)  LinearizeAsGain=on  AntiWindupMode=clamping  Kb=1  LimitIntegrator=off  UpperIntegratorSaturationLimit=inf  LowerIntegratorSaturationLimit=-inf  PGainOutDataTypeStr=single  PProdOutDataTypeStr=single  POutMin=[]  POutMax=[]  IGainOutDataTypeStr=single  IProdOutDataTypeStr=single  IOutMin=[]  IOutMax=[]  DOutMin=[]  DOutMax=[]  NOutMin=[]  NOutMax=[]  SumOutDataTypeStr=single  SumOutMin=[]  SumOutMax=[]  SaturationOutDataTypeStr=single  SaturationOutMin=[]  SaturationOutMax=[]  PParamMin=[]  PParamMax=[]  IParamMin=[]  IParamMax=[]  DParamMin=[]  DParamMax=[]  NParamMin=[]  NParamMax=[]  KbParamMin=[]  KbParamMax=[]  KtParamMin=[]  KtParamMax=[]  KbOutMin=[]  KbOutMax=[]  KtOutMin=[]  KtOutMax=[]  IntegratorOutMin=[]  IntegratorOutMax=[]  FilterOutMin=[]  FilterOutMax=[]  SumI1OutMin=[]  SumI1OutMax=[]  SumI2OutMin=[]  SumI2OutMax=[]  SumI3OutMin=[]  SumI3OutMax=[]  SumI4OutMin=[]  SumI4OutMax=[]  SumDOutMin=[]  SumDOutMax=[]  DifferentiatorOutMin=[]  DifferentiatorOutMax=[]  FilterDiffOutCoefMin=[]  FilterDiffOutCoefMax=[]  ReciprocalOutMin=[]  ReciprocalOutMax=[]  SumDenOutMin=[]  SumDenOutMax=[]  SumNumOutMin=[]  SumNumOutMax=[]  DivideOutMin=[]  DivideOutMax=[]  UdiffTsProdOutMin=[]  UdiffTsProdOutMax=[]  NTsProdOutMin=[]  NTsProdOutMax=[]  UintegralTsProdOutMin=[]  UintegralTsProdOutMax=[]  UngainTsProdOutMin=[]  UngainTsProdOutMax=[]  ClampingZeroOutDataTypeStr=Inherit: Inherit via back propagation  ClampingZeroOutMin=[]  ClampingZeroOutMax=[]  FilterDenConstantOutDataTypeStr=Inherit: Inherit via back propagation  FilterDenConstantOutMin=[]  FilterDenConstantOutMax=[]  PCopyOutDataTypeStr=Inherit: Inherit via back propagation  PCopyOutMin=[]  PCopyOutMax=[]  NCopyOutDataTypeStr=Inherit: Inherit via back propagation  NCopyOutMin=[]  NCopyOutMax=[]  IntegratorContinuousStateAttributes=''  IntegratorStateMustResolveToSignalObject=off  IntegratorRTWStateStorageClass=Auto  FilterContinuousStateAttributes=''  FilterStateMustResolveToSignalObject=off  FilterRTWStateStorageClass=Auto  ParallelPVariant=ExternalParameters  IdealPVariant=Disabled  IVariant=ExternalParameters  DVariant=Disabled  IntegratorVariant=Discrete  SatVariant=Enabled  AWVariant=DiscClampingParallel  PCopyVariant=Disabled  TRVariant=Disabled  FdbkBlocksVariant=Forward  IdealPFdbkVariant=Disabled  SatFdbkVariant=Disabled  DerivativeFilterVariant=Disabled  NVariant=Disabled  NCopyVariant=Disabled_SignalSpec  FilterICVariant=Disabled  IntegratorICVariant=InternalICs  ExternalResetVariant=Disabled  TRSumVariant=Passthrough  SumFdbkVariant=Disabled  SumVariant=Sum_PI  TsampFilterVariant=InternalTs  TsampNgainVariant=Passthrough  TsampIntegralVariant=Disabled_SignalSpec  ExternalSaturationOutDataTypeStr=Inherit: Same as second input
  Scope : Scope  NumInputPorts=2
  Sum1 : Sum  Inputs=|+-  OutDataTypeStr=single  AccumDataTypeStr=single
  Sum7 : Sum  Inputs=|+-  OutDataTypeStr=single  AccumDataTypeStr=single
  ud_ref : Outport  OutDataTypeStr=single
  uq_ref : Outport  Port=2  OutDataTypeStr=single
  wires:
  id_fdbk/1 -> Sum1/2
  Constant/1 -> Sum1/1
  iq_fdbk/1 -> Sum7/2
  Sum1/1 -> PID Controller1/1
  Sum7/1 -> PID Controller2/1
  PID Controller1/1 -> Scope/1, ud_ref/1
  PID Controller2/1 -> Scope/2, uq_ref/1
  iq_ref/1 -> Sum7/1
  Constant3/1 -> PID Controller1/2
  Constant4/1 -> PID Controller1/3
  Constant1/1 -> PID Controller2/2
  Constant2/1 -> PID Controller2/3

== system PMSM_NFLUX_v1_0/FOC/current_loop/Nonlinear Flux Observer/LPF ==
  note: [LPF formula]
      | we(k)=we(k-1)+LPF_K*(wm(k)-we(k-1))
      | wm=Omega/Pn*30/pi
  obs_wm : Inport  OutDataTypeStr=single  PortDimensions=1
  LPFFilter : Constant  Value=LPF_K  OutDataTypeStr=single
  err : Sum  Inputs=+-
  sum : Sum
  x : Product
  z1 : UnitDelay  InitialCondition=single(0)  SampleTime=-1  HasFrameUpgradeWarning=on
  we : Outport  OutDataTypeStr=single
  wires:
  obs_wm/1 -> err/1
  z1/1 -> sum/2, err/2
  x/1 -> sum/1
  sum/1 -> z1/1, we/1
  LPFFilter/1 -> x/1
  err/1 -> x/2

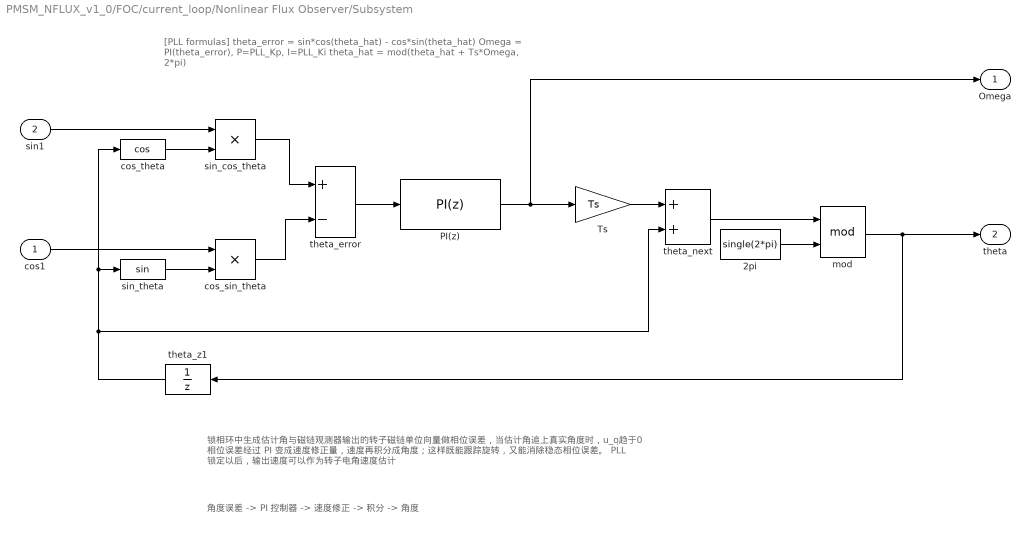
== system PMSM_NFLUX_v1_0/FOC/current_loop/Nonlinear Flux Observer/Subsystem ==
  note: 角度误差 -> PI 控制器 -> 速度修正 -> 积分 -> 角度
  note: 锁相环中生成估计角与磁链观测器输出的转子磁链单位向量做相位误差，当估计角追上真实角度时，u_q趋于0
      | 相位误差经过 PI 变成速度修正量，速度再积分成角度；这样既能跟踪旋转，又能消除稳态相位误差。
      | PLL 锁定以后，输出速度可以作为转子电角速度估计
  note: [PLL formulas]
      | theta_error = sin*cos(theta_hat) - cos*sin(theta_hat)
      | Omega = PI(theta_error),  P=PLL_Kp,  I=PLL_Ki
      | theta_hat = mod(theta_hat + Ts*Omega, 2*pi)
  cos1 : Inport  OutDataTypeStr=single  PortDimensions=1
  sin1 : Inport  Port=2  OutDataTypeStr=single  PortDimensions=1
  2pi : Constant  Value=single(2*pi)  OutDataTypeStr=single
  PI(z) : slpidlib/PID Controller  Controller=PI  Form=Parallel  TimeDomain=Discrete-time  UseExternalTs=off  SampleTime=-1  IntegratorMethod=Forward Euler  FilterMethod=Forward Euler  ControllerParametersSource=internal  P=PLL_Kp  I=PLL_Ki  UseKiTs=off  D=0  N=100  UseFilter=on  TunerSelectOption=Transfer Function Based (PID Tuner App)  InitialConditionSource=internal  InitialConditionForIntegrator=0  InitialConditionForFilter=0  DifferentiatorICPrevScaledInput=0  ExternalReset=none  TrackingMode=off  Kt=1  LimitOutput=on  SatLimitsSource=internal  UpperSaturationLimit=PLL_OmegaLimit  LowerSaturationLimit=-PLL_OmegaLimit  LinearizeAsGain=off  AntiWindupMode=none  Kb=1  LimitIntegrator=off  UpperIntegratorSaturationLimit=inf  LowerIntegratorSaturationLimit=-inf  POutMin=[]  POutMax=[]  IOutMin=[]  IOutMax=[]  DOutMin=[]  DOutMax=[]  NOutMin=[]  NOutMax=[]  SumOutMin=[]  SumOutMax=[]  SaturationOutMin=[]  SaturationOutMax=[]  PParamMin=[]  PParamMax=[]  IParamMin=[]  IParamMax=[]  DParamMin=[]  DParamMax=[]  NParamMin=[]  NParamMax=[]  KbParamMin=[]  KbParamMax=[]  KtParamMin=[]  KtParamMax=[]  KbOutMin=[]  KbOutMax=[]  KtOutMin=[]  KtOutMax=[]  IntegratorOutMin=[]  IntegratorOutMax=[]  FilterOutMin=[]  FilterOutMax=[]  SumI1OutMin=[]  SumI1OutMax=[]  SumI2OutMin=[]  SumI2OutMax=[]  SumI3OutMin=[]  SumI3OutMax=[]  SumI4OutMin=[]  SumI4OutMax=[]  SumDOutMin=[]  SumDOutMax=[]  DifferentiatorOutMin=[]  DifferentiatorOutMax=[]  FilterDiffOutCoefMin=[]  FilterDiffOutCoefMax=[]  ReciprocalOutMin=[]  ReciprocalOutMax=[]  SumDenOutMin=[]  SumDenOutMax=[]  SumNumOutMin=[]  SumNumOutMax=[]  DivideOutMin=[]  DivideOutMax=[]  UdiffTsProdOutMin=[]  UdiffTsProdOutMax=[]  NTsProdOutMin=[]  NTsProdOutMax=[]  UintegralTsProdOutMin=[]  UintegralTsProdOutMax=[]  UngainTsProdOutMin=[]  UngainTsProdOutMax=[]  ClampingZeroOutDataTypeStr=Inherit: Inherit via back propagation  ClampingZeroOutMin=[]  ClampingZeroOutMax=[]  FilterDenConstantOutDataTypeStr=Inherit: Inherit via back propagation  FilterDenConstantOutMin=[]  FilterDenConstantOutMax=[]  PCopyOutDataTypeStr=Inherit: Inherit via back propagation  PCopyOutMin=[]  PCopyOutMax=[]  NCopyOutDataTypeStr=Inherit: Inherit via back propagation  NCopyOutMin=[]  NCopyOutMax=[]  IntegratorContinuousStateAttributes=''  IntegratorStateMustResolveToSignalObject=off  IntegratorRTWStateStorageClass=Auto  FilterContinuousStateAttributes=''  FilterStateMustResolveToSignalObject=off  FilterRTWStateStorageClass=Auto  ParallelPVariant=InternalParameters  IdealPVariant=Disabled  IVariant=InternalParameters  DVariant=Disabled  IntegratorVariant=Discrete  SatVariant=Enabled  AWVariant=Passthrough  PCopyVariant=Disabled  TRVariant=Disabled  FdbkBlocksVariant=Forward  IdealPFdbkVariant=Disabled  SatFdbkVariant=Disabled  DerivativeFilterVariant=Disabled  NVariant=Disabled  NCopyVariant=Disabled_SignalSpec  FilterICVariant=Disabled  IntegratorICVariant=InternalICs  ExternalResetVariant=Disabled  TRSumVariant=Passthrough  SumFdbkVariant=Disabled  SumVariant=Sum_PI  TsampFilterVariant=InternalTs  TsampNgainVariant=Passthrough  TsampIntegralVariant=Disabled_SignalSpec  ExternalSaturationOutDataTypeStr=Inherit: Same as second input
      settings: LibrarySourceBlock=simulink/Discrete/Discrete PID Controller
  Ts : Gain  Gain=Ts
  cos_sin_theta : Product
  cos_theta : Trigonometry  Operator=cos
  mod : Math  Operator=mod
  sin_cos_theta : Product
  sin_theta : Trigonometry
  theta_error : Sum  Inputs=+-
  theta_next : Sum
  theta_z1 : UnitDelay  InitialCondition=single(0)  SampleTime=-1  HasFrameUpgradeWarning=on
  Omega : Outport  OutDataTypeStr=single
  theta : Outport  Port=2  OutDataTypeStr=single
  wires:
  mod/1 -> theta/1, theta_z1/1
  Ts/1 -> theta_next/1
  cos1/1 -> cos_sin_theta/1
  theta_z1/1 -> cos_theta/1, sin_theta/1, theta_next/2
  sin_theta/1 -> cos_sin_theta/2
  2pi/1 -> mod/2
  theta_error/1 -> PI(z)/1
  cos_sin_theta/1 -> theta_error/2
  PI(z)/1 -> Omega/1, Ts/1
  cos_theta/1 -> sin_cos_theta/2
  sin_cos_theta/1 -> theta_error/1
  theta_next/1 -> mod/1
  sin1/1 -> sin_cos_theta/1

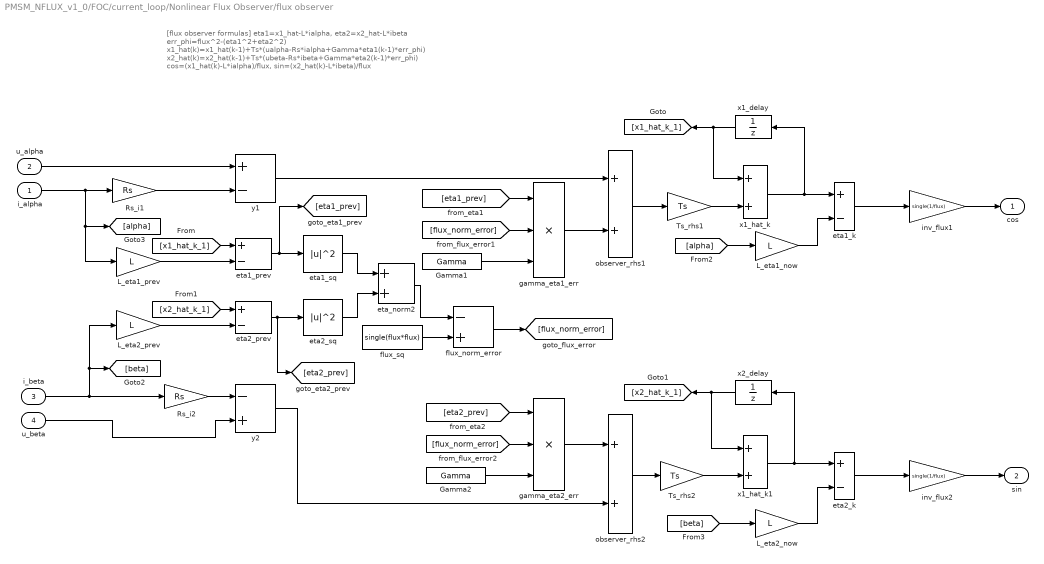
== system PMSM_NFLUX_v1_0/FOC/current_loop/Nonlinear Flux Observer/flux observer ==
  note: [flux observer formulas]
      | eta1=x1_hat-L*ialpha, eta2=x2_hat-L*ibeta
      | err_phi=flux^2-(eta1^2+eta2^2)
      | x1_hat(k)=x1_hat(k-1)+Ts*(ualpha-Rs*ialpha+Gamma*eta1(k-1)*err_phi)
      | x2_hat(k)=x2_hat(k-1)+Ts*(ubeta-Rs*ibeta+Gamma*eta2(k-1)*err_phi)
      | cos=(x1_hat(k)-L*ialpha)/flux, sin=(x2_hat(k)-L*ibeta)/flux
  i_alpha : Inport  OutDataTypeStr=single  PortDimensions=1
  u_alpha : Inport  Port=2  OutDataTypeStr=single  PortDimensions=1
  i_beta : Inport  Port=3  OutDataTypeStr=single  PortDimensions=1
  u_beta : Inport  Port=4  OutDataTypeStr=single  PortDimensions=1
  Gamma1 : Constant  Value=Gamma  OutDataTypeStr=single
  Gamma2 : Constant  Value=Gamma  OutDataTypeStr=single
  L_eta1_now : Gain  Gain=L
  L_eta1_prev : Gain  Gain=L
  L_eta2_now : Gain  Gain=L
  L_eta2_prev : Gain  Gain=L
  Rs_i1 : Gain  Gain=Rs
  Rs_i2 : Gain  Gain=Rs
  Ts_rhs1 : Gain  Gain=Ts
  Ts_rhs2 : Gain  Gain=Ts
  eta1_k : Sum  Inputs=+-
  eta1_prev : Sum  Inputs=+-
  eta1_sq : Math  Operator=magnitude^2
  eta2_k : Sum  Inputs=+-
  eta2_prev : Sum  Inputs=+-
  eta2_sq : Math  Operator=magnitude^2
  eta_norm2 : Sum
  flux_norm_error : Sum  Inputs=-+
  flux_sq : Constant  Value=single(flux*flux)  OutDataTypeStr=single
  gamma_eta1_err : Product  Inputs=***
  gamma_eta2_err : Product  Inputs=***
  inv_flux1 : Gain  Gain=single(1/flux)
  inv_flux2 : Gain  Gain=single(1/flux)
  observer_rhs1 : Sum
  observer_rhs2 : Sum
  x1_delay : UnitDelay  InitialCondition=single(0)  SampleTime=-1  HasFrameUpgradeWarning=on
  x1_hat_k : Sum
  x1_hat_k1 : Sum
  x2_delay : UnitDelay  InitialCondition=single(0)  SampleTime=-1  HasFrameUpgradeWarning=on
  y1 : Sum  Inputs=+-
  y2 : Sum  Inputs=-+
  cos : Outport  OutDataTypeStr=single
  sin : Outport  Port=2  OutDataTypeStr=single
  wires:
  [eta2_prev] -> gamma_eta2_err/1
  Rs_i1/1 -> y1/2
  Gamma1/1 -> gamma_eta1_err/3
  eta1_sq/1 -> eta_norm2/1
  eta1_k/1 -> inv_flux1/1
  Ts_rhs1/1 -> x1_hat_k/2
  eta2_prev/1 -> eta2_sq/1, [eta2_prev]
  Rs_i2/1 -> y2/1
  [flux_norm_error] -> gamma_eta1_err/2
  flux_norm_error/1 -> [flux_norm_error]
  L_eta2_prev/1 -> eta2_prev/2
  eta2_k/1 -> inv_flux2/1
  x1_hat_k1/1 -> eta2_k/1, x2_delay/1
  i_alpha/1 -> L_eta1_prev/1, [alpha], Rs_i1/1
  x2_delay/1 -> [x2_hat_k_1], x1_hat_k1/1
  [x1_hat_k_1] -> eta1_prev/1
  eta1_prev/1 -> eta1_sq/1, [eta1_prev]
  [flux_norm_error] -> gamma_eta2_err/2
  u_alpha/1 -> y1/1
  eta_norm2/1 -> flux_norm_error/1
  x1_hat_k/1 -> eta1_k/1, x1_delay/1
  i_beta/1 -> [beta], L_eta2_prev/1, Rs_i2/1
  [alpha] -> L_eta1_now/1
  y1/1 -> observer_rhs1/1
  observer_rhs2/1 -> Ts_rhs2/1
  [eta1_prev] -> gamma_eta1_err/1
  observer_rhs1/1 -> Ts_rhs1/1
  inv_flux2/1 -> sin/1
  x1_delay/1 -> [x1_hat_k_1], x1_hat_k/1
  L_eta2_now/1 -> eta2_k/2
  L_eta1_prev/1 -> eta1_prev/2
  [x2_hat_k_1] -> eta2_prev/1
  flux_sq/1 -> flux_norm_error/2
  eta2_sq/1 -> eta_norm2/2
  y2/1 -> observer_rhs2/2
  gamma_eta2_err/1 -> observer_rhs2/1
  inv_flux1/1 -> cos/1
  Gamma2/1 -> gamma_eta2_err/3
  u_beta/1 -> y2/2
  gamma_eta1_err/1 -> observer_rhs1/2
  Ts_rhs2/1 -> x1_hat_k1/2
  [beta] -> L_eta2_now/1
  L_eta1_now/1 -> eta1_k/2

== system PMSM_NFLUX_v1_0/FOC/current_loop/SVPWM/InvClark ==
  Valpha : Inport  OutDataTypeStr=single
  Vbeta : Inport  Port=2  OutDataTypeStr=single
  Gain : Gain  Gain=-1/2  OutDataTypeStr=single
  Gain1 : Gain  Gain=sqrt(3)/2  OutDataTypeStr=single
  Sum : Sum  Inputs=|++  OutDataTypeStr=single
  Sum1 : Sum  Inputs=-+|  OutDataTypeStr=single
  Va : Outport  OutDataTypeStr=single
  Vb : Outport  Port=2  OutDataTypeStr=single
  Vc : Outport  Port=3  OutDataTypeStr=single
  wires:
  Valpha/1 -> Gain/1, Va/1
  Vbeta/1 -> Gain1/1
  Gain/1 -> Sum1/2, Sum/1
  Sum/1 -> Vb/1
  Gain1/1 -> Sum1/1, Sum/2
  Sum1/1 -> Vc/1

== system PMSM_NFLUX_v1_0/FOC/current_loop/SVPWM/ei_t ==
  Vabc : Inport  OutDataTypeStr=single
  Demux : Demux  Outputs=3
  Gain : Gain  Gain=-1/2  OutDataTypeStr=single
  Min : MinMax  Inputs=3  OutDataTypeStr=single
  Min1 : MinMax  Function=max  Inputs=3  OutDataTypeStr=single
  Sum : Sum  Inputs=|++  OutDataTypeStr=single
  ei_t : Outport  OutDataTypeStr=single
  wires:
  Min/1 -> Sum/1
  Sum/1 -> Gain/1
  Min1/1 -> Sum/2
  Gain/1 -> ei_t/1
  Vabc/1 -> Demux/1
  Demux/1 -> Min1/1, Min/1
  Demux/2 -> Min/2, Min1/2
  Demux/3 -> Min1/3, Min/3
